simulink model "CE141IntroModel1"  (R2014b)
settings: Solver=ode45  StartTime=0.0  StopTime=20  MaxStep=0.1  RelTol=1e-3
settings Model: Creator=Dejan  LastModifiedBy=Dejan
settings DataIOCC: SignalLoggingSaveFormat=ModelDataLogs
settings OptimizationCC: ExpressionDepthLimit=2147483647
settings DebuggingCC: UnderspecifiedInitializationDetection=Classic  MergeDetectMultiDrivingBlocksExec=none  SolverPrmCheckMsg=none  FcnCallInpInsideContextMsg=EnableAllAsWarning  StateNameClashWarn=warning
settings GRTTargetCC: CombineOutputUpdateFcns=off  GRTInterface=on

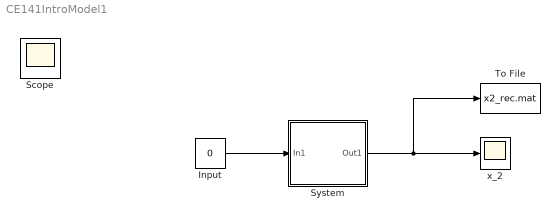
== system CE141IntroModel1 ==
  Input : Constant  Value=0
  System : Subsystem
  To File : ToFile  Filename=x2_rec.mat  MatrixName=x2_rec  SaveFormat=Timeseries
  x_2 : Scope
      settings: TimeRange=4  YMin=-3.65625  YMax=0.3437500000000004
  Scope : Scope
      settings: MaxDataPoints=7500
  wires:
  System/1(Out1) -> x_2/1, To File/1
  Input/1 -> System/1(In1)

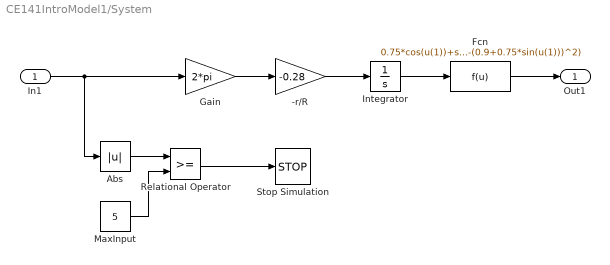
== system CE141IntroModel1/System ==
  In1 : Inport
  -r/R : Gain  Gain=-0.28
  Abs : Abs
  Fcn : Fcn  Expr=0.75*cos(u(1))+sqrt(4.8^2-(0.9+0.75*sin(u(1)))^2)
  Gain : Gain  Gain=2*pi
  Integrator : Integrator  InitialCondition=1
  MaxInput : Constant  Value=5
  Relational Operator : RelationalOperator  OutDataTypeStr=boolean
  Stop Simulation : Stop
  Out1 : Outport
  wires:
  Integrator/1 -> Fcn/1
  Fcn/1 -> Out1/1
  Gain/1 -> -r/R/1
  -r/R/1 -> Integrator/1
  Relational Operator/1 -> Stop Simulation/1
  In1/1 -> Abs/1, Gain/1
  Abs/1 -> Relational Operator/1
  MaxInput/1 -> Relational Operator/2
